simulink model "Rotating_panels"  (R2024b)
settings: Solver=VariableStepAuto  StartTime=0.0  StopTime=10.0  RelTol=1e-3
undefined symbols (not defined in the file): J, Kd, Kf, Kg, L, V
settings Model: Creator=Administrator  LastModifiedBy=saibot

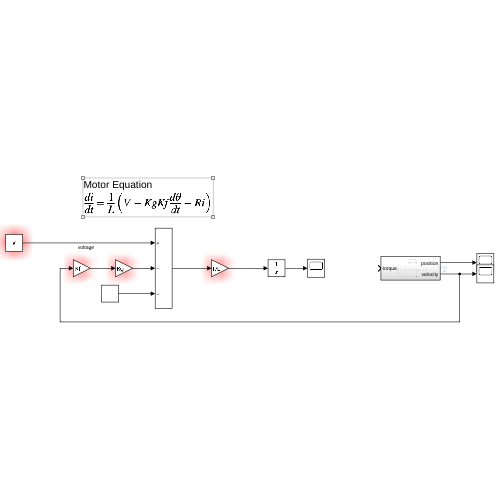
[thumbnail: Simulink's stored preview of the top-level diagram]
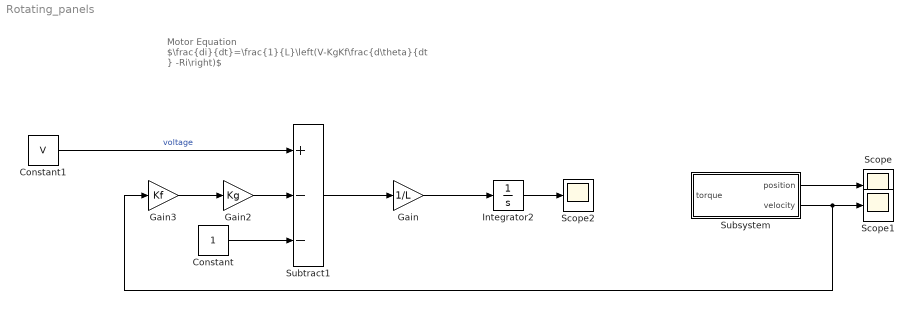
== system Rotating_panels ==
  note: Motor Equation
      | $\frac{di}{dt}=\frac{1}{L}\left(V-KgKf\frac{d\theta}{dt } -Ri\right)$
  Constant : Constant
  Constant1 : Constant  Value=V
  Gain : Gain  Gain=1/L
  Gain2 : Gain  Gain=Kg
  Gain3 : Gain  Gain=Kf
  Integrator2 : Integrator
  Scope : Scope
  Scope1 : Scope
  Scope2 : Scope
  Subsystem : Subsystem
  Subtract1 : Sum  Inputs=+--
  wires:
  Subsystem/1(position) -> Scope/1
  Subsystem/2(velocity) -> Gain3/1, Scope1/1
  Gain3/1 -> Gain2/1
  Gain2/1 -> Subtract1/2
  Constant1/1 -> Subtract1/1  "voltage"
  Gain/1 -> Integrator2/1
  Subtract1/1 -> Gain/1
  Constant/1 -> Subtract1/3
  Integrator2/1 -> Scope2/1

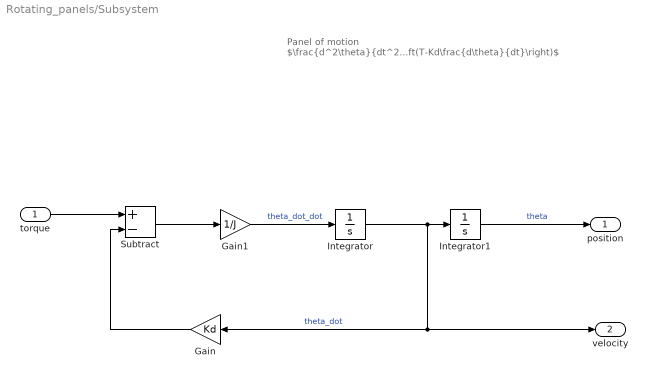
== system Rotating_panels/Subsystem ==
  note: Panel of motion
      |
      | $\frac{d^2\theta}{dt^2}=\frac{1}{J}\left(T-Kd\frac{d\theta}{dt}\right)$
  torque : Inport
  Gain : Gain  Gain=Kd
  Gain1 : Gain  Gain=1/J
  Integrator : Integrator
  Integrator1 : Integrator
  Subtract : Sum  Inputs=+-
  position : Outport
  velocity : Outport  Port=2
  wires:
  torque/1 -> Subtract/1
  Subtract/1 -> Gain1/1
  Integrator/1 -> Integrator1/1, velocity/1, Gain/1  "theta_dot"
  Integrator1/1 -> position/1  "theta"
  Gain1/1 -> Integrator/1  "theta_dot_dot"
  Gain/1 -> Subtract/2
